simulink model "Myp5NLOpenLoopObserver"  (R2021b)
settings: Solver=ode4  StartTime=0.0  StopTime=TIME_SIM  FixedStep=STEP_SIZE  MaxStep=Ts  RelTol=1e-6
values from neighbouring files (symbols this model uses):
  Dd = [0  0; 0  0.0001229087]    [LinearModel.mat]
  v_OP = 20    [LinearModel.mat]
  xOP = [1.2671 122.9087 0.00454800621385]    [LinearModel.mat]
undefined symbols (not defined in the file or in its folder): Area, Bd, beta_OP, Cc0, CP, CP0, Ff, Gg, Jg, Jr, Kd, L, Lambda_legend, Ng, Pe_rated, Pitch_legend, R, rho_air, Tg_OP, Ts
libraries: simulink_extras x2
settings Model: Creator=roga  LastModifiedBy=tanzc
settings SolverCC: AlgebraicLoopSolver=TrustRegion
settings DataIOCC: SaveFinalState=on  SaveFormat=Array  ReturnWorkspaceOutputs=off
settings OptimizationCC: LifeSpan=inf
settings DebuggingCC: UnderspecifiedInitializationDetection=Classic  MergeDetectMultiDrivingBlocksExec=none  SolverPrmCheckMsg=warning  StateNameClashWarn=warning  SFUnexpectedBacktrackingDiag=warning  SFNoUnconditionalDefaultTransitionDiag=warning  SFExecutionAtInitializationDiag=none  SFMachineParentedDataDiag=warning  ArithmeticOperatorsInVariantConditions=warning
settings HardwareCC: ProdBitPerPointer=32  ProdBitPerSizeT=32  ProdBitPerPtrDiffT=32  ProdLargestAtomicFloat=None  ProdIntDivRoundTo=Undefined  ProdEndianess=Unspecified  ProdWordSize=32  ProdHWDeviceType=32-bit Generic
settings ModelReferenceCC: PropagateSignalLabelsOutOfModel=off
settings SFSimCC: SimUseLocalCustomCode=off  CustomCodeUndefinedFunction=UseInterfaceOnly
settings RTWCC: RTWUseLocalCustomCode=off
settings CodeAppCC: StateflowObjectComments=on
settings GRTTargetCC: TargetLangStandard=C89/C90 (ANSI)
settings ConfigComp: CovMetricSettings=dw  CovSaveCumulativeToWorkspaceVar=on  CovSaveSingleToWorkspaceVar=on  CovExternalEMLEnable=off

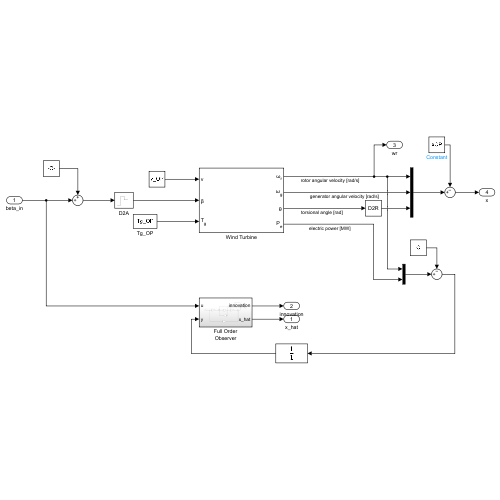
[thumbnail: Simulink's stored preview of the top-level diagram]
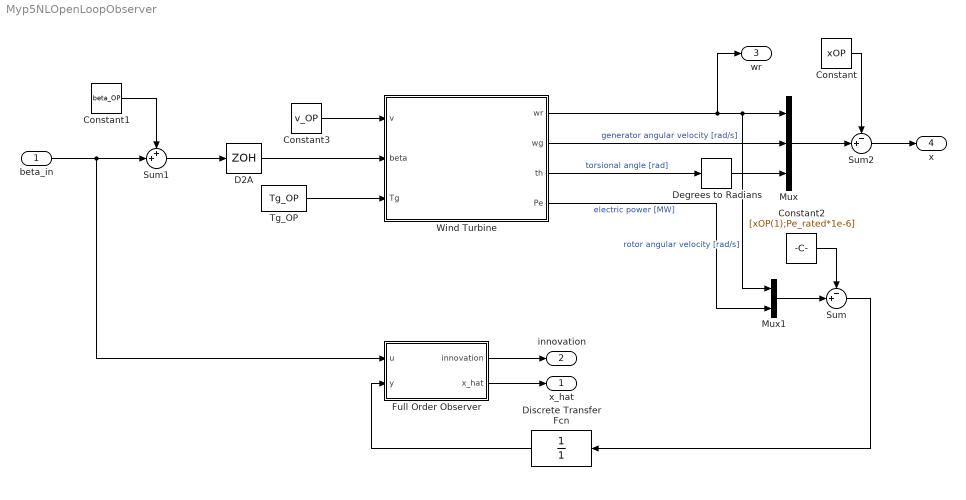
== system Myp5NLOpenLoopObserver ==
  beta_in : Inport
  Constant : Constant  Value=xOP
  Constant1 : Constant  Value=beta_OP  SampleTime=Ts
  Constant2 : Constant  Value=[xOP(1);Pe_rated*1e-6]
  Constant3 : Constant  Value=v_OP
  D2A : ZeroOrderHold  SampleTime=-1
  Degrees to Radians : simulink_extras/Transformations/Degrees to Radians
  Discrete Transfer Fcn : DiscreteTransferFcn  Denominator=1  SampleTime=Ts
  Full Order Observer : Subsystem
  Mux : Mux  Inputs=3
  Mux1 : Mux  Inputs=2
  Sum : Sum  Inputs=-+|
  Sum1 : Sum  Inputs=++|
  Sum2 : Sum  Inputs=-+|
  Tg_OP : Constant  Value=Tg_OP
  Wind Turbine : Subsystem
      mask Display:
      | port_label('input',1,'v')
      | port_label('input',2,'\beta','Interpreter','tex')
      | port_label('input',3,'T_g','Interpreter','tex')
      | port_label('output',1,'\omega_r','Interpreter','tex')
      | port_label('output',2,'\omega_g','Interpreter','tex')
      | port_label('output',3,'\theta','Interpreter','tex')
      | port_label('output',4,'P_e','Interpreter','tex')
  x_hat : Outport
  innovation : Outport  Port=2
  wr : Outport  Port=3
  x : Outport  Port=4
  wires:
  Wind Turbine/2(wg) -> Mux/2  "generator angular velocity [rad/s]"
  Wind Turbine/4(Pe) -> Mux1/2  "electric power [MW]"
  Constant3/1 -> Wind Turbine/1(v)
  Tg_OP/1 -> Wind Turbine/3(Tg)
  Wind Turbine/3(th) -> Degrees to Radians/1  "torsional angle [rad]"
  D2A/1 -> Wind Turbine/2(beta)
  Wind Turbine/1(wr) -> Mux1/1, Mux/1, wr/1  "rotor angular velocity [rad/s]"
  Full Order Observer/2(x_hat) -> x_hat/1
  Full Order Observer/1(innovation) -> innovation/1
  Mux1/1 -> Sum/2
  Sum1/1 -> D2A/1
  Constant1/1 -> Sum1/1
  Constant2/1 -> Sum/1
  Sum/1 -> Discrete Transfer Fcn/1
  Discrete Transfer Fcn/1 -> Full Order Observer/2(y)
  Degrees to Radians/1 -> Mux/3
  Mux/1 -> Sum2/2
  Constant/1 -> Sum2/1
  Sum2/1 -> x/1
  beta_in/1 -> Full Order Observer/1(u), Sum1/2

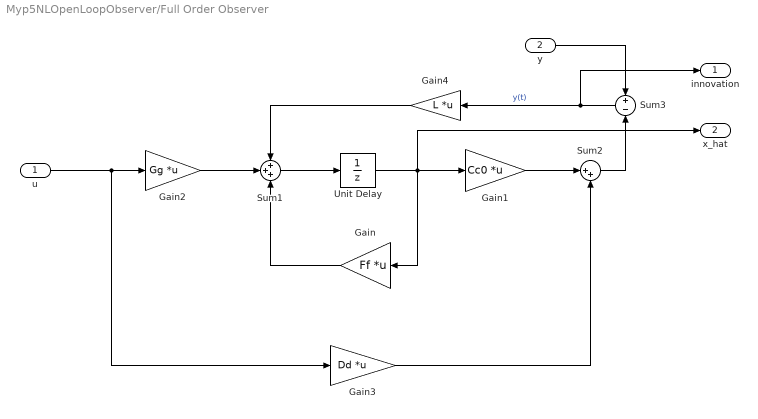
== system Myp5NLOpenLoopObserver/Full Order Observer ==
  u : Inport
  y : Inport  Port=2
  Gain : Gain  Gain=Ff  Multiplication=Matrix(K*u) (u vector)
  Gain1 : Gain  Gain=Cc0  Multiplication=Matrix(K*u) (u vector)
  Gain2 : Gain  Gain=Gg  Multiplication=Matrix(K*u) (u vector)
  Gain3 : Gain  Gain=Dd  Multiplication=Matrix(K*u) (u vector)
  Gain4 : Gain  Gain=L  Multiplication=Matrix(K*u) (u vector)
  Sum1 : Sum  Inputs=+++
  Sum2 : Sum  Inputs=|++
  Sum3 : Sum  Inputs=+-
  Unit Delay : UnitDelay  SampleTime=Ts  HasFrameUpgradeWarning=on
  innovation : Outport
  x_hat : Outport  Port=2
  wires:
  y/1 -> Sum3/1
  Gain1/1 -> Sum2/1
  Unit Delay/1 -> x_hat/1, Gain/1, Gain1/1
  Gain2/1 -> Sum1/2
  Sum2/1 -> Sum3/2
  u/1 -> Gain3/1, Gain2/1
  Gain3/1 -> Sum2/2
  Gain/1 -> Sum1/3
  Gain4/1 -> Sum1/1
  Sum1/1 -> Unit Delay/1
  Sum3/1 -> innovation/1, Gain4/1  "y(t)"

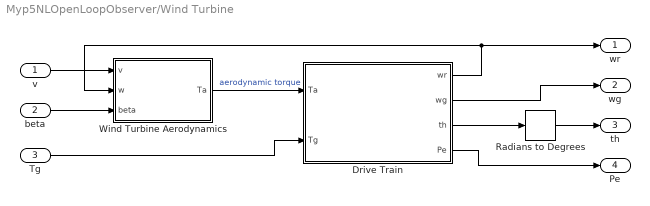
== system Myp5NLOpenLoopObserver/Wind Turbine ==
  v : Inport
  beta : Inport  Port=2
  Tg : Inport  Port=3
  Drive Train : Subsystem
      mask Display:
      | port_label('input',1,'T_a','Interpreter','tex')
      | port_label('input',2,'T_g','Interpreter','tex')
      | port_label('output',1,'\omega_r','Interpreter','tex')
      | port_label('output',2,'\omega_g','Interpreter','tex')
      | port_label('output',3,'\theta','Interpreter','tex')
      | port_label('output',4,'P_e','Interpreter','tex')
  Radians to Degrees : simulink_extras/Transformations/Radians to Degrees
  Wind Turbine Aerodynamics : Subsystem
      mask Display:
      | port_label('input',1,'v')
      | port_label('input',2,'\omega_r','Interpreter','tex')
      | port_label('input',3,'\beta','Interpreter','tex')
      | port_label('output',1,'T_a','Interpreter','tex')
  wr : Outport  VectorParamsAs1DForOutWhenUnconnected=off
  wg : Outport  Port=2  VectorParamsAs1DForOutWhenUnconnected=off
  th : Outport  Port=3  VectorParamsAs1DForOutWhenUnconnected=off
  Pe : Outport  Port=4  VectorParamsAs1DForOutWhenUnconnected=off
  wires:
  Drive Train/1(wr) -> wr/1, Wind Turbine Aerodynamics/2(w)
  Tg/1 -> Drive Train/2(Tg)
  Drive Train/2(wg) -> wg/1
  Drive Train/4(Pe) -> Pe/1
  beta/1 -> Wind Turbine Aerodynamics/3(beta)
  Wind Turbine Aerodynamics/1(Ta) -> Drive Train/1(Ta)  "aerodynamic torque"
  v/1 -> Wind Turbine Aerodynamics/1(v)
  Drive Train/3(th) -> Radians to Degrees/1
  Radians to Degrees/1 -> th/1

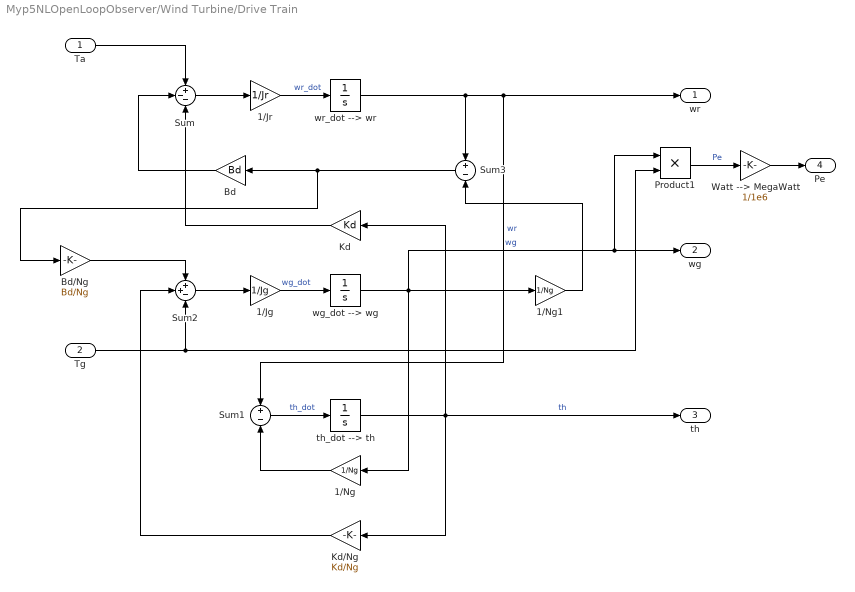
== system Myp5NLOpenLoopObserver/Wind Turbine/Drive Train ==
  Ta : Inport
  Tg : Inport  Port=2
  1/Jg : Gain  Gain=1/Jg
  1/Jr : Gain  Gain=1/Jr
  1/Ng : Gain  Gain=1/Ng
  1/Ng1 : Gain  Gain=1/Ng
  Bd : Gain  Gain=Bd
  Bd/Ng : Gain  Gain=Bd/Ng
  Kd : Gain  Gain=Kd
  Kd/Ng : Gain  Gain=Kd/Ng
  Product1 : Product
  Sum : Sum  Inputs=+--
  Sum1 : Sum  Inputs=+-
  Sum2 : Sum  Inputs=++-
  Sum3 : Sum  Inputs=+-
  Watt --> MegaWatt : Gain  Gain=1/1e6
  th_dot --> th : Integrator  Priority=3  InitialCondition=xOP(3)  LowerSaturationLimit=0
  wg_dot --> wg : Integrator  Priority=2  InitialCondition=xOP(2)  LowerSaturationLimit=0
  wr_dot --> wr : Integrator  Priority=1  InitialCondition=xOP(1)  LowerSaturationLimit=0
  wr : Outport  VectorParamsAs1DForOutWhenUnconnected=off
  wg : Outport  Port=2  VectorParamsAs1DForOutWhenUnconnected=off
  th : Outport  Port=3  VectorParamsAs1DForOutWhenUnconnected=off
  Pe : Outport  Port=4  VectorParamsAs1DForOutWhenUnconnected=off
  wires:
  wg_dot --> wg/1 -> Product1/1, wg/1, 1/Ng1/1, 1/Ng/1  "wg"
  wr_dot --> wr/1 -> Sum3/1, wr/1, Sum1/1  "wr"
  1/Ng/1 -> Sum1/2
  Sum1/1 -> th_dot --> th/1  "th_dot"
  Sum2/1 -> 1/Jg/1
  1/Ng1/1 -> Sum3/2
  Sum/1 -> 1/Jr/1
  1/Jr/1 -> wr_dot --> wr/1  "wr_dot"
  th_dot --> th/1 -> th/1, Kd/Ng/1, Kd/1  "th"
  1/Jg/1 -> wg_dot --> wg/1  "wg_dot"
  Sum3/1 -> Bd/Ng/1, Bd/1
  Bd/1 -> Sum/2
  Kd/1 -> Sum/3
  Bd/Ng/1 -> Sum2/1
  Kd/Ng/1 -> Sum2/2
  Ta/1 -> Sum/1
  Tg/1 -> Product1/2, Sum2/3
  Product1/1 -> Watt --> MegaWatt/1  "Pe"
  Watt --> MegaWatt/1 -> Pe/1

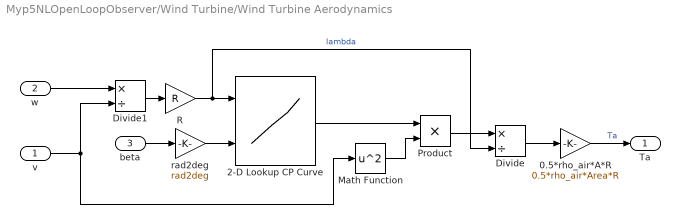
== system Myp5NLOpenLoopObserver/Wind Turbine/Wind Turbine Aerodynamics ==
  v : Inport
  w : Inport  Port=2
  beta : Inport  Port=3
  0.5*rho_air*A*R : Gain  Gain=0.5*rho_air*Area*R
  2-D Lookup CP Curve : Lookup_n-D  BreakpointsForDimension1=Lambda_legend  BreakpointsForDimension2=Pitch_legend  BreakpointsForDimension3=CP0'  Table=CP  DiagnosticForOutOfRangeInput=Warning  RndMeth=Simplest  InputSameDT=on
      settings: InputPortMap=u0,u1
  Divide : Product  Inputs=*/
  Divide1 : Product  Inputs=*/
  Math Function : Math  Operator=square  SignedPower=on  SaturateOnIntegerOverflow=on
  Product : Product
  R : Gain  Gain=R
  rad2deg : Gain  Gain=rad2deg
  Ta : Outport  VectorParamsAs1DForOutWhenUnconnected=off
  wires:
  0.5*rho_air*A*R/1 -> Ta/1  "Ta"
  beta/1 -> rad2deg/1
  w/1 -> Divide1/1
  Divide/1 -> 0.5*rho_air*A*R/1
  Product/1 -> Divide/1
  Math Function/1 -> Product/2
  2-D Lookup CP Curve/1 -> Product/1
  v/1 -> Divide1/2, Math Function/1
  Divide1/1 -> R/1
  R/1 -> Divide/2, 2-D Lookup CP Curve/1  "lambda"
  rad2deg/1 -> 2-D Lookup CP Curve/2
